simulink model "FSAC2021"  (R2014a)
settings: Solver=FixedStepDiscrete  StartTime=0.0  StopTime=inf  FixedStep=0.0005  RelTol=1e-3
model workspace (MAT data in the model file):
  MCOS : class17 (value not decoded)
  MCOS : class17 (value not decoded)
  MCOS : class17 (value not decoded)
  MCOS : class17 (value not decoded)
  MCOS : class17 (value not decoded)
  MCOS : class17 (value not decoded)
  MCOS : class17 (value not decoded)
  MCOS : class17 (value not decoded)
  MCOS : class17 (value not decoded)
  MCOS : class17 (value not decoded)
  MCOS : class17 (value not decoded)
  MCOS : class17 (value not decoded)
  MCOS : class17 (value not decoded)
  MCOS : class17 (value not decoded)
  MCOS : class17 (value not decoded)
  MCOS : class17 (value not decoded)
  MCOS : class17 (value not decoded)
  MCOS : class17 (value not decoded)
  MCOS : class17 (value not decoded)
  BUZZER_START = 1
  MCOS : class17 (value not decoded)
  MCOS : class17 (value not decoded)
  MCOS : class17 (value not decoded)
  MCOS : class17 (value not decoded)
  MCOS : class17 (value not decoded)
  MCOS : class17 (value not decoded)
  MCOS : class17 (value not decoded)
  MCOS : class17 (value not decoded)
  MCOS : class17 (value not decoded)
  MCOS : class17 (value not decoded)
  MCOS : class17 (value not decoded)
  MCOS : class17 (value not decoded)
  MCOS : class17 (value not decoded)
  MCOS : class17 (value not decoded)
  MCOS : class17 (value not decoded)
  MCOS : class17 (value not decoded)
  MCOS : class17 (value not decoded)
  MCOS : class17 (value not decoded)
  MCOS : class17 (value not decoded)
  MCOS : class17 (value not decoded)
  MCOS : class17 (value not decoded)
  MCOS : class17 (value not decoded)
  MCOS : class17 (value not decoded)
  MCOS : class17 (value not decoded)
  MCOS : class17 (value not decoded)
  MCOS : class17 (value not decoded)
  MCOS : class17 (value not decoded)
  MCOS : class17 (value not decoded)
  MCOS : class17 (value not decoded)
  MCOS : class17 (value not decoded)
  MCOS : class17 (value not decoded)
  MCOS : class17 (value not decoded)
  MCOS : class17 (value not decoded)
  MCOS : class17 (value not decoded)
  MCOS : class17 (value not decoded)
  MCOS : class17 (value not decoded)
  MCOS : class17 (value not decoded)
  MCOS : class17 (value not decoded)
  Brake = 11
  MCOS : class17 (value not decoded)
  MCOS : class17 (value not decoded)
  MCOS : class17 (value not decoded)
  MCOS : class17 (value not decoded)
  MCOS : class17 (value not decoded)
  MCOS : class17 (value not decoded)
  MCOS : class17 (value not decoded)
  MCOS : class17 (value not decoded)
  Sensor_Acc_b = 101.85
  Sensor_Acc_k = -0.0185
  Str_Sen_Orig_Angle = -341
  MCOS : class17 (value not decoded)
  Tire_D = 0.47
  T = 0.05
libraries: simulink x396, ec55xxlib x126
(part 6 of 17)

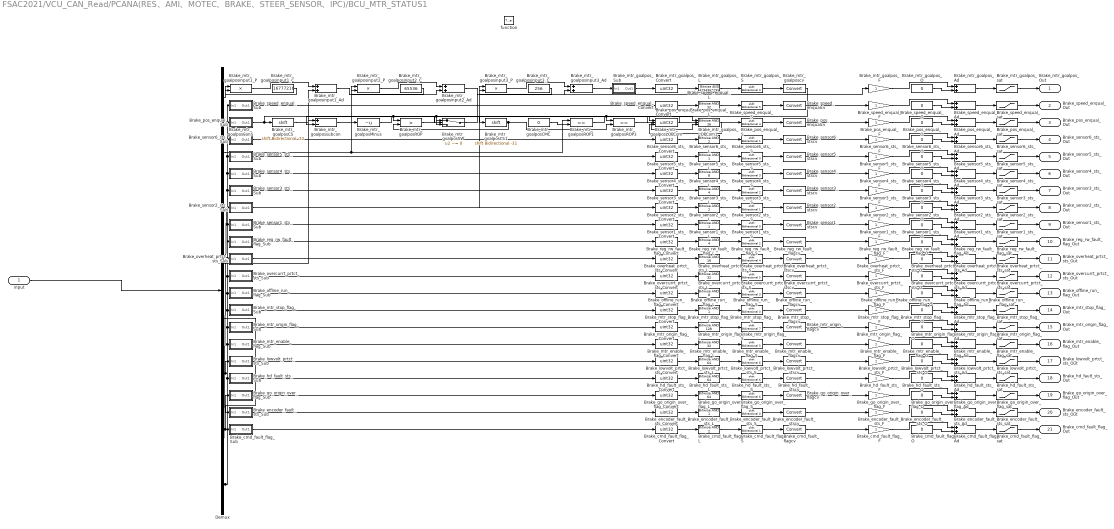
== system FSAC2021/VCU_CAN_Read/PCANA(RES、AMI、MOTEC、BRAKE、STEER_SENSOR、IPC)/BCU_MTR_STATUS1 ==
  input : Inport
  function : TriggerPort  TriggerType=function-call
  Brake_cmd_fault_flag_Ad : Sum
  Brake_cmd_fault_flag_Convert : DataTypeConversion  OutDataTypeStr=uint32
  Brake_cmd_fault_flag_F : Gain
  Brake_cmd_fault_flag_L : simulink/Logic and Bit Operations/Bitwise Operator  logicop=AND  UseBitMask=on  BitMask=2  BitMaskRealWorld=Stored Integer
  Brake_cmd_fault_flag_O : Constant  Value=0  OutDataTypeStr=single
  Brake_cmd_fault_flag_S : ArithShift  BitShiftNumber=1
  Brake_cmd_fault_flag_Sub : Subsystem
  Brake_cmd_fault_flag_sat : Saturate  UpperLimit=1  LowerLimit=0
  Brake_cmd_fault_flagcv : DataTypeConversion
  Brake_encoder_fault_sts_Ad : Sum
  Brake_encoder_fault_sts_Convert : DataTypeConversion  OutDataTypeStr=uint32
  Brake_encoder_fault_sts_F : Gain
  Brake_encoder_fault_sts_L : simulink/Logic and Bit Operations/Bitwise Operator  logicop=AND  UseBitMask=on  BitMask=1  BitMaskRealWorld=Stored Integer
  Brake_encoder_fault_sts_O : Constant  Value=0  OutDataTypeStr=single
  Brake_encoder_fault_sts_S : ArithShift
  Brake_encoder_fault_sts_Sub : Subsystem
  Brake_encoder_fault_sts_sat : Saturate  UpperLimit=1  LowerLimit=0
  Brake_encoder_fault_stscv : DataTypeConversion
  Brake_go_origin_over_flag_Ad : Sum
  Brake_go_origin_over_flag_Convert : DataTypeConversion  OutDataTypeStr=uint32
  Brake_go_origin_over_flag_F : Gain
  Brake_go_origin_over_flag_L : simulink/Logic and Bit Operations/Bitwise Operator  logicop=AND  UseBitMask=on  BitMask=64  BitMaskRealWorld=Stored Integer
  Brake_go_origin_over_flag_O : Constant  Value=0  OutDataTypeStr=single
  Brake_go_origin_over_flag_S : ArithShift  BitShiftNumber=6
  Brake_go_origin_over_flag_Sub : Subsystem
  Brake_go_origin_over_flag_sat : Saturate  UpperLimit=1  LowerLimit=0
  Brake_go_origin_over_flagcv : DataTypeConversion
  Brake_hd_fault_sts_Ad : Sum
  Brake_hd_fault_sts_Convert : DataTypeConversion  OutDataTypeStr=uint32
  Brake_hd_fault_sts_F : Gain
  Brake_hd_fault_sts_L : simulink/Logic and Bit Operations/Bitwise Operator  logicop=AND  UseBitMask=on  BitMask=64  BitMaskRealWorld=Stored Integer
  Brake_hd_fault_sts_O : Constant  Value=0  OutDataTypeStr=single
  Brake_hd_fault_sts_S : ArithShift  BitShiftNumber=6
  Brake_hd_fault_sts_Sub : Subsystem
  Brake_hd_fault_sts_sat : Saturate  UpperLimit=1  LowerLimit=0
  Brake_hd_fault_stscv : DataTypeConversion
  Brake_lowvolt_prtct_sts_Ad : Sum
  Brake_lowvolt_prtct_sts_Convert : DataTypeConversion  OutDataTypeStr=uint32
  Brake_lowvolt_prtct_sts_F : Gain
  Brake_lowvolt_prtct_sts_L : simulink/Logic and Bit Operations/Bitwise Operator  logicop=AND  UseBitMask=on  BitMask=64  BitMaskRealWorld=Stored Integer
  Brake_lowvolt_prtct_sts_O : Constant  Value=0  OutDataTypeStr=single
  Brake_lowvolt_prtct_sts_S : ArithShift  BitShiftNumber=6
  Brake_lowvolt_prtct_sts_Sub : Subsystem
  Brake_lowvolt_prtct_sts_sat : Saturate  UpperLimit=1  LowerLimit=0
  Brake_lowvolt_prtct_stscv : DataTypeConversion
  Brake_mtr_enable_flag_Ad : Sum
  Brake_mtr_enable_flag_Convert : DataTypeConversion  OutDataTypeStr=uint32
  Brake_mtr_enable_flag_F : Gain
  Brake_mtr_enable_flag_L : simulink/Logic and Bit Operations/Bitwise Operator  logicop=AND  UseBitMask=on  BitMask=32  BitMaskRealWorld=Stored Integer
  Brake_mtr_enable_flag_O : Constant  Value=0  OutDataTypeStr=single
  Brake_mtr_enable_flag_S : ArithShift  BitShiftNumber=5
  Brake_mtr_enable_flag_Sub : Subsystem
  Brake_mtr_enable_flag_sat : Saturate  UpperLimit=1  LowerLimit=0
  Brake_mtr_enable_flagcv : DataTypeConversion
  Brake_mtr_goalposCMC : Constant  Value=0
  Brake_mtr_goalposCS : ArithShift  BitShiftNumber=-32
  Brake_mtr_goalposCS1 : ArithShift  BitShiftNumber=-31
  Brake_mtr_goalposConS : Constant  OutDataTypeStr=single
  Brake_mtr_goalposLOPCom : Logic  Operator=OR  AllPortsSameDT=off  OutDataTypeStr=boolean
  Brake_mtr_goalposMinus : UnaryMinus
  Brake_mtr_goalposROP : RelationalOperator  Operator=>  OutDataTypeStr=boolean
  Brake_mtr_goalposROP1 : RelationalOperator  Operator===  OutDataTypeStr=boolean
  Brake_mtr_goalposROP3 : RelationalOperator  Operator===  OutDataTypeStr=boolean
  Brake_mtr_goalposSW : Switch  Criteria=u2 ~= 0
  Brake_mtr_goalpos_Ad : Sum
  Brake_mtr_goalpos_Convert : DataTypeConversion  OutDataTypeStr=uint32
  Brake_mtr_goalpos_F : Gain
  Brake_mtr_goalpos_L : simulink/Logic and Bit Operations/Bitwise Operator  logicop=AND  UseBitMask=on  BitMask=4294967295  BitMaskRealWorld=Stored Integer
  Brake_mtr_goalpos_LOPCom1 : Logic  AllPortsSameDT=off  OutDataTypeStr=boolean
  Brake_mtr_goalpos_O : Constant  Value=0  OutDataTypeStr=single
  Brake_mtr_goalpos_S : ArithShift
  Brake_mtr_goalpos_Sub : Subsystem
  Brake_mtr_goalpos_sat : Saturate  UpperLimit=2147483647  LowerLimit=-2147483648
  Brake_mtr_goalposcv : DataTypeConversion
  Brake_mtr_goalposinput1_Ad : Sum
  Brake_mtr_goalposinput1_C : Constant  Value=16777216
  Brake_mtr_goalposinput1_P : Product
  Brake_mtr_goalposinput2_Ad : Sum
  Brake_mtr_goalposinput2_C : Constant  Value=65536
  Brake_mtr_goalposinput2_P : Product
  Brake_mtr_goalposinput3_Ad : Sum
  Brake_mtr_goalposinput3_C : Constant  Value=256
  Brake_mtr_goalposinput3_P : Product
  Brake_mtr_goalpossubcon : Sum  Inputs=+-
  Brake_mtr_origin_flag_Ad : Sum
  Brake_mtr_origin_flag_Convert : DataTypeConversion  OutDataTypeStr=uint32
  Brake_mtr_origin_flag_F : Gain
  Brake_mtr_origin_flag_L : simulink/Logic and Bit Operations/Bitwise Operator  logicop=AND  UseBitMask=on  BitMask=128  BitMaskRealWorld=Stored Integer
  Brake_mtr_origin_flag_O : Constant  Value=0  OutDataTypeStr=single
  Brake_mtr_origin_flag_S : ArithShift  BitShiftNumber=7
  Brake_mtr_origin_flag_Sub : Subsystem
  Brake_mtr_origin_flag_sat : Saturate  UpperLimit=1  LowerLimit=0
  Brake_mtr_origin_flagcv : DataTypeConversion
  Brake_mtr_stop_flag_Ad : Sum
  Brake_mtr_stop_flag_Convert : DataTypeConversion  OutDataTypeStr=uint32
  Brake_mtr_stop_flag_F : Gain
  Brake_mtr_stop_flag_L : simulink/Logic and Bit Operations/Bitwise Operator  logicop=AND  UseBitMask=on  BitMask=1  BitMaskRealWorld=Stored Integer
  Brake_mtr_stop_flag_O : Constant  Value=0  OutDataTypeStr=single
  Brake_mtr_stop_flag_S : ArithShift
  Brake_mtr_stop_flag_Sub : Subsystem
  Brake_mtr_stop_flag_sat : Saturate  UpperLimit=1  LowerLimit=0
  Brake_mtr_stop_flagcv : DataTypeConversion
  Brake_offline_run_flag_Ad : Sum
  Brake_offline_run_flag_Convert : DataTypeConversion  OutDataTypeStr=uint32
  Brake_offline_run_flag_F : Gain
  Brake_offline_run_flag_L : simulink/Logic and Bit Operations/Bitwise Operator  logicop=AND  UseBitMask=on  BitMask=8  BitMaskRealWorld=Stored Integer
  Brake_offline_run_flag_O : Constant  Value=0  OutDataTypeStr=single
  Brake_offline_run_flag_S : ArithShift  BitShiftNumber=3
  Brake_offline_run_flag_Sub : Subsystem
  Brake_offline_run_flag_sat : Saturate  UpperLimit=1  LowerLimit=0
  Brake_offline_run_flagcv : DataTypeConversion
  Brake_overcurrt_prtct_sts_Ad : Sum
  Brake_overcurrt_prtct_sts_Convert : DataTypeConversion  OutDataTypeStr=uint32
  Brake_overcurrt_prtct_sts_F : Gain
  Brake_overcurrt_prtct_sts_L : simulink/Logic and Bit Operations/Bitwise Operator  logicop=AND  UseBitMask=on  BitMask=32  BitMaskRealWorld=Stored Integer
  Brake_overcurrt_prtct_sts_O : Constant  Value=0  OutDataTypeStr=single
  Brake_overcurrt_prtct_sts_S : ArithShift  BitShiftNumber=5
  Brake_overcurrt_prtct_sts_Sub : Subsystem
  Brake_overcurrt_prtct_sts_sat : Saturate  UpperLimit=1  LowerLimit=0
  Brake_overcurrt_prtct_stscv : DataTypeConversion
  Brake_overheat_prtct_sts_Ad : Sum
  Brake_overheat_prtct_sts_Convert : DataTypeConversion  OutDataTypeStr=uint32
  Brake_overheat_prtct_sts_F : Gain
  Brake_overheat_prtct_sts_L : simulink/Logic and Bit Operations/Bitwise Operator  logicop=AND  UseBitMask=on  BitMask=16  BitMaskRealWorld=Stored Integer
  Brake_overheat_prtct_sts_O : Constant  Value=0  OutDataTypeStr=single
  Brake_overheat_prtct_sts_S : ArithShift  BitShiftNumber=4
  Brake_overheat_prtct_sts_Sub : Subsystem
  Brake_overheat_prtct_sts_sat : Saturate  UpperLimit=1  LowerLimit=0
  Brake_overheat_prtct_stscv : DataTypeConversion
  Brake_pos_enqual_Ad : Sum
  Brake_pos_enqual_Convert : DataTypeConversion  OutDataTypeStr=uint32
  Brake_pos_enqual_F : Gain
  Brake_pos_enqual_L : simulink/Logic and Bit Operations/Bitwise Operator  logicop=AND  UseBitMask=on  BitMask=16  BitMaskRealWorld=Stored Integer
  Brake_pos_enqual_O : Constant  Value=0  OutDataTypeStr=single
  Brake_pos_enqual_S : ArithShift  BitShiftNumber=4
  Brake_pos_enqual_Sub : Subsystem
  Brake_pos_enqual_sat : Saturate  UpperLimit=1  LowerLimit=0
  Brake_pos_enqualcv : DataTypeConversion
  Brake_reg_rw_fault_flag_Ad : Sum
  Brake_reg_rw_fault_flag_Convert : DataTypeConversion  OutDataTypeStr=uint32
  Brake_reg_rw_fault_flag_F : Gain
  Brake_reg_rw_fault_flag_L : simulink/Logic and Bit Operations/Bitwise Operator  logicop=AND  UseBitMask=on  BitMask=4  BitMaskRealWorld=Stored Integer
  Brake_reg_rw_fault_flag_O : Constant  Value=0  OutDataTypeStr=single
  Brake_reg_rw_fault_flag_S : ArithShift  BitShiftNumber=2
  Brake_reg_rw_fault_flag_Sub : Subsystem
  Brake_reg_rw_fault_flag_sat : Saturate  UpperLimit=1  LowerLimit=0
  Brake_reg_rw_fault_flagcv : DataTypeConversion
  Brake_sensor1_sts_Ad : Sum
  Brake_sensor1_sts_Convert : DataTypeConversion  OutDataTypeStr=uint32
  Brake_sensor1_sts_F : Gain
  Brake_sensor1_sts_L : simulink/Logic and Bit Operations/Bitwise Operator  logicop=AND  UseBitMask=on  BitMask=1  BitMaskRealWorld=Stored Integer
  Brake_sensor1_sts_O : Constant  Value=0  OutDataTypeStr=single
  Brake_sensor1_sts_S : ArithShift
  Brake_sensor1_sts_Sub : Subsystem
  Brake_sensor1_sts_sat : Saturate  UpperLimit=1  LowerLimit=0
  Brake_sensor1_stscv : DataTypeConversion
  Brake_sensor2_sts_Ad : Sum
  Brake_sensor2_sts_Convert : DataTypeConversion  OutDataTypeStr=uint32
  Brake_sensor2_sts_F : Gain
  Brake_sensor2_sts_L : simulink/Logic and Bit Operations/Bitwise Operator  logicop=AND  UseBitMask=on  BitMask=2  BitMaskRealWorld=Stored Integer
  Brake_sensor2_sts_O : Constant  Value=0  OutDataTypeStr=single
  Brake_sensor2_sts_S : ArithShift  BitShiftNumber=1
  Brake_sensor2_sts_Sub : Subsystem
  Brake_sensor2_sts_sat : Saturate  UpperLimit=1  LowerLimit=0
  Brake_sensor2_stscv : DataTypeConversion
  Brake_sensor3_sts_Ad : Sum
  Brake_sensor3_sts_Convert : DataTypeConversion  OutDataTypeStr=uint32
  Brake_sensor3_sts_F : Gain
  Brake_sensor3_sts_L : simulink/Logic and Bit Operations/Bitwise Operator  logicop=AND  UseBitMask=on  BitMask=4  BitMaskRealWorld=Stored Integer
  Brake_sensor3_sts_O : Constant  Value=0  OutDataTypeStr=single
  Brake_sensor3_sts_S : ArithShift  BitShiftNumber=2
  Brake_sensor3_sts_Sub : Subsystem
  Brake_sensor3_sts_sat : Saturate  UpperLimit=1  LowerLimit=0
  Brake_sensor3_stscv : DataTypeConversion
  Brake_sensor4_sts_Ad : Sum
  Brake_sensor4_sts_Convert : DataTypeConversion  OutDataTypeStr=uint32
  Brake_sensor4_sts_F : Gain
  Brake_sensor4_sts_L : simulink/Logic and Bit Operations/Bitwise Operator  logicop=AND  UseBitMask=on  BitMask=8  BitMaskRealWorld=Stored Integer
  Brake_sensor4_sts_O : Constant  Value=0  OutDataTypeStr=single
  Brake_sensor4_sts_S : ArithShift  BitShiftNumber=3
  Brake_sensor4_sts_Sub : Subsystem
  Brake_sensor4_sts_sat : Saturate  UpperLimit=1  LowerLimit=0
  Brake_sensor4_stscv : DataTypeConversion
  Brake_sensor5_sts_Ad : Sum
  Brake_sensor5_sts_Convert : DataTypeConversion  OutDataTypeStr=uint32
  Brake_sensor5_sts_F : Gain
  Brake_sensor5_sts_L : simulink/Logic and Bit Operations/Bitwise Operator  logicop=AND  UseBitMask=on  BitMask=1  BitMaskRealWorld=Stored Integer
  Brake_sensor5_sts_O : Constant  Value=0  OutDataTypeStr=single
  Brake_sensor5_sts_S : ArithShift
  Brake_sensor5_sts_Sub : Subsystem
  Brake_sensor5_sts_sat : Saturate  UpperLimit=1  LowerLimit=0
  Brake_sensor5_stscv : DataTypeConversion
  Brake_sensor6_sts_Ad : Sum
  Brake_sensor6_sts_Convert : DataTypeConversion  OutDataTypeStr=uint32
  Brake_sensor6_sts_F : Gain
  Brake_sensor6_sts_L : simulink/Logic and Bit Operations/Bitwise Operator  logicop=AND  UseBitMask=on  BitMask=2  BitMaskRealWorld=Stored Integer
  Brake_sensor6_sts_O : Constant  Value=0  OutDataTypeStr=single
  Brake_sensor6_sts_S : ArithShift  BitShiftNumber=1
  Brake_sensor6_sts_Sub : Subsystem
  Brake_sensor6_sts_sat : Saturate  UpperLimit=1  LowerLimit=0
  Brake_sensor6_stscv : DataTypeConversion
  Brake_speed_enqual_Ad : Sum
  Brake_speed_enqual_Convert : DataTypeConversion  OutDataTypeStr=uint32
  Brake_speed_enqual_F : Gain
  Brake_speed_enqual_L : simulink/Logic and Bit Operations/Bitwise Operator  logicop=AND  UseBitMask=on  BitMask=32  BitMaskRealWorld=Stored Integer
  Brake_speed_enqual_O : Constant  Value=0  OutDataTypeStr=single
  Brake_speed_enqual_S : ArithShift  BitShiftNumber=5
  Brake_speed_enqual_Sub : Subsystem
  Brake_speed_enqual_sat : Saturate  UpperLimit=1  LowerLimit=0
  Brake_speed_enqualcv : DataTypeConversion
  Demux : Demux  Outputs=8
  Brake_mtr_goalpos_Out : Outport
  Brake_speed_enqual_Out : Outport  Port=2
  Brake_pos_enqual_Out : Outport  Port=3
  Brake_sensor6_sts_Out : Outport  Port=4
  Brake_sensor5_sts_Out : Outport  Port=5
  Brake_sensor4_sts_Out : Outport  Port=6
  Brake_sensor3_sts_Out : Outport  Port=7
  Brake_sensor2_sts_Out : Outport  Port=8
  Brake_sensor1_sts_Out : Outport  Port=9
  Brake_reg_rw_fault_flag_Out : Outport  Port=10
  Brake_overheat_prtct_sts_Out : Outport  Port=11
  Brake_overcurrt_prtct_sts_Out : Outport  Port=12
  Brake_offline_run_flag_Out : Outport  Port=13
  Brake_mtr_stop_flag_Out : Outport  Port=14
  Brake_mtr_origin_flag_Out : Outport  Port=15
  Brake_mtr_enable_flag_Out : Outport  Port=16
  Brake_lowvolt_prtct_sts_Out : Outport  Port=17
  Brake_hd_fault_sts_Out : Outport  Port=18
  Brake_go_origin_over_flag_Out : Outport  Port=19
  Brake_encoder_fault_sts_Out : Outport  Port=20
  Brake_cmd_fault_flag_Out : Outport  Port=21
  wires:
  Brake_mtr_goalpos_F/1 -> Brake_mtr_goalpos_Ad/1
  Brake_mtr_goalpos_O/1 -> Brake_mtr_goalpos_Ad/2
  Brake_mtr_goalpos_Ad/1 -> Brake_mtr_goalpos_sat/1
  Brake_mtr_goalpos_sat/1 -> Brake_mtr_goalpos_Out/1
  Demux/1 -> Brake_mtr_goalposinput1_P/1
  Brake_mtr_goalposinput1_C/1 -> Brake_mtr_goalposinput1_P/2
  Brake_mtr_goalposinput1_P/1 -> Brake_mtr_goalposinput1_Ad/1
  Demux/4 -> Brake_mtr_goalposinput1_Ad/2
  Demux/2 -> Brake_mtr_goalposinput2_P/1, Brake_mtr_goalposROP1/1
  Brake_mtr_goalposinput2_C/1 -> Brake_mtr_goalposinput2_P/2
  Brake_mtr_goalposinput2_P/1 -> Brake_mtr_goalposinput2_Ad/1
  Brake_mtr_goalposinput1_Ad/1 -> Brake_mtr_goalposinput2_Ad/2
  Demux/3 -> Brake_mtr_goalposinput3_P/1
  Brake_mtr_goalposinput3_C/1 -> Brake_mtr_goalposinput3_P/2
  Brake_mtr_goalposinput3_P/1 -> Brake_mtr_goalposinput3_Ad/1
  Brake_mtr_goalposinput2_Ad/1 -> Brake_mtr_goalposinput3_Ad/2
  Brake_mtr_goalposinput3_Ad/1 -> Brake_mtr_goalpos_Sub/1(In1)
  Brake_mtr_goalpos_Sub/1(Out1) -> Brake_mtr_goalpos_Convert/1
  Brake_mtr_goalpos_Convert/1 -> Brake_mtr_goalpos_L/1
  Brake_mtr_goalpos_L/1 -> Brake_mtr_goalpos_S/1
  Brake_mtr_goalpos_S/1 -> Brake_mtr_goalposcv/1
  Brake_mtr_goalposcv/1 -> Brake_mtr_goalposROP/1, Brake_mtr_goalpossubcon/2, Brake_mtr_goalposSW/3, Brake_mtr_goalposROP3/1
  Brake_mtr_goalposConS/1 -> Brake_mtr_goalposCS/1, Brake_mtr_goalposCS1/1
  Brake_mtr_goalposCS1/1 -> Brake_mtr_goalposROP/2, Brake_mtr_goalposROP3/2
  Brake_mtr_goalposCS/1 -> Brake_mtr_goalpossubcon/1
  Brake_mtr_goalpossubcon/1 -> Brake_mtr_goalposMinus/1
  Brake_mtr_goalposMinus/1 -> Brake_mtr_goalposSW/1
  Brake_mtr_goalposSW/1 -> Brake_mtr_goalpos_F/1
  Brake_mtr_goalposROP1/1 -> Brake_mtr_goalpos_LOPCom1/1
  Brake_mtr_goalposROP3/1 -> Brake_mtr_goalpos_LOPCom1/2
  Brake_mtr_goalpos_LOPCom1/1 -> Brake_mtr_goalposLOPCom/2
  Brake_mtr_goalposROP/1 -> Brake_mtr_goalposLOPCom/1
  Brake_mtr_goalposLOPCom/1 -> Brake_mtr_goalposSW/2
  Brake_mtr_goalposCMC/1 -> Brake_mtr_goalposROP1/2
  Brake_speed_enqual_F/1 -> Brake_speed_enqual_Ad/1
  Brake_speed_enqual_O/1 -> Brake_speed_enqual_Ad/2
  Brake_speed_enqual_Ad/1 -> Brake_speed_enqual_sat/1
  Brake_speed_enqual_sat/1 -> Brake_speed_enqual_Out/1
  Demux/8 -> Brake_speed_enqual_Sub/1(In1), Brake_pos_enqual_Sub/1(In1), Brake_sensor4_sts_Sub/1(In1), Brake_sensor3_sts_Sub/1(In1), Brake_sensor1_sts_Sub/1(In1), Brake_mtr_origin_flag_Sub/1(In1), Brake_hd_fault_sts_Sub/1(In1), Brake_sensor2_sts_Sub/1(In1)
  Brake_speed_enqual_Sub/1(Out1) -> Brake_speed_enqual_Convert/1
  Brake_speed_enqual_Convert/1 -> Brake_speed_enqual_L/1
  Brake_speed_enqual_L/1 -> Brake_speed_enqual_S/1
  Brake_speed_enqual_S/1 -> Brake_speed_enqualcv/1
  Brake_speed_enqualcv/1 -> Brake_speed_enqual_F/1
  Brake_pos_enqual_F/1 -> Brake_pos_enqual_Ad/1
  Brake_pos_enqual_O/1 -> Brake_pos_enqual_Ad/2
  Brake_pos_enqual_Ad/1 -> Brake_pos_enqual_sat/1
  Brake_pos_enqual_sat/1 -> Brake_pos_enqual_Out/1
  Brake_pos_enqual_Sub/1(Out1) -> Brake_pos_enqual_Convert/1
  Brake_pos_enqual_Convert/1 -> Brake_pos_enqual_L/1
  Brake_pos_enqual_L/1 -> Brake_pos_enqual_S/1
  Brake_pos_enqual_S/1 -> Brake_pos_enqualcv/1
  Brake_pos_enqualcv/1 -> Brake_pos_enqual_F/1
  Brake_sensor6_sts_F/1 -> Brake_sensor6_sts_Ad/1
  Brake_sensor6_sts_O/1 -> Brake_sensor6_sts_Ad/2
  Brake_sensor6_sts_Ad/1 -> Brake_sensor6_sts_sat/1
  Brake_sensor6_sts_sat/1 -> Brake_sensor6_sts_Out/1
  Demux/6 -> Brake_sensor6_sts_Sub/1(In1), Brake_sensor5_sts_Sub/1(In1), Brake_overheat_prtct_sts_Sub/1(In1), Brake_overcurrt_prtct_sts_Sub/1(In1), Brake_lowvolt_prtct_sts_Sub/1(In1)
  Brake_sensor6_sts_Sub/1(Out1) -> Brake_sensor6_sts_Convert/1
  Brake_sensor6_sts_Convert/1 -> Brake_sensor6_sts_L/1
  Brake_sensor6_sts_L/1 -> Brake_sensor6_sts_S/1
  Brake_sensor6_sts_S/1 -> Brake_sensor6_stscv/1
  Brake_sensor6_stscv/1 -> Brake_sensor6_sts_F/1
  Brake_sensor5_sts_F/1 -> Brake_sensor5_sts_Ad/1
  Brake_sensor5_sts_O/1 -> Brake_sensor5_sts_Ad/2
  Brake_sensor5_sts_Ad/1 -> Brake_sensor5_sts_sat/1
  Brake_sensor5_sts_sat/1 -> Brake_sensor5_sts_Out/1
  Brake_sensor5_sts_Sub/1(Out1) -> Brake_sensor5_sts_Convert/1
  Brake_sensor5_sts_Convert/1 -> Brake_sensor5_sts_L/1
  Brake_sensor5_sts_L/1 -> Brake_sensor5_sts_S/1
  Brake_sensor5_sts_S/1 -> Brake_sensor5_stscv/1
  Brake_sensor5_stscv/1 -> Brake_sensor5_sts_F/1
  Brake_sensor4_sts_F/1 -> Brake_sensor4_sts_Ad/1
  Brake_sensor4_sts_O/1 -> Brake_sensor4_sts_Ad/2
  Brake_sensor4_sts_Ad/1 -> Brake_sensor4_sts_sat/1
  Brake_sensor4_sts_sat/1 -> Brake_sensor4_sts_Out/1
  Brake_sensor4_sts_Sub/1(Out1) -> Brake_sensor4_sts_Convert/1
  Brake_sensor4_sts_Convert/1 -> Brake_sensor4_sts_L/1
  Brake_sensor4_sts_L/1 -> Brake_sensor4_sts_S/1
  Brake_sensor4_sts_S/1 -> Brake_sensor4_stscv/1
  Brake_sensor4_stscv/1 -> Brake_sensor4_sts_F/1
  Brake_sensor3_sts_F/1 -> Brake_sensor3_sts_Ad/1
  Brake_sensor3_sts_O/1 -> Brake_sensor3_sts_Ad/2
  Brake_sensor3_sts_Ad/1 -> Brake_sensor3_sts_sat/1
  Brake_sensor3_sts_sat/1 -> Brake_sensor3_sts_Out/1
  Brake_sensor3_sts_Sub/1(Out1) -> Brake_sensor3_sts_Convert/1
  Brake_sensor3_sts_Convert/1 -> Brake_sensor3_sts_L/1
  Brake_sensor3_sts_L/1 -> Brake_sensor3_sts_S/1
  Brake_sensor3_sts_S/1 -> Brake_sensor3_stscv/1
  Brake_sensor3_stscv/1 -> Brake_sensor3_sts_F/1
  Brake_sensor2_sts_F/1 -> Brake_sensor2_sts_Ad/1
  Brake_sensor2_sts_O/1 -> Brake_sensor2_sts_Ad/2
  Brake_sensor2_sts_Ad/1 -> Brake_sensor2_sts_sat/1
  Brake_sensor2_sts_sat/1 -> Brake_sensor2_sts_Out/1
  Brake_sensor2_sts_Sub/1(Out1) -> Brake_sensor2_sts_Convert/1
  Brake_sensor2_sts_Convert/1 -> Brake_sensor2_sts_L/1
  Brake_sensor2_sts_L/1 -> Brake_sensor2_sts_S/1
  Brake_sensor2_sts_S/1 -> Brake_sensor2_stscv/1
  Brake_sensor2_stscv/1 -> Brake_sensor2_sts_F/1
  Brake_sensor1_sts_F/1 -> Brake_sensor1_sts_Ad/1
  Brake_sensor1_sts_O/1 -> Brake_sensor1_sts_Ad/2
  Brake_sensor1_sts_Ad/1 -> Brake_sensor1_sts_sat/1
  Brake_sensor1_sts_sat/1 -> Brake_sensor1_sts_Out/1
  Brake_sensor1_sts_Sub/1(Out1) -> Brake_sensor1_sts_Convert/1
  Brake_sensor1_sts_Convert/1 -> Brake_sensor1_sts_L/1
  Brake_sensor1_sts_L/1 -> Brake_sensor1_sts_S/1
  Brake_sensor1_sts_S/1 -> Brake_sensor1_stscv/1
  Brake_sensor1_stscv/1 -> Brake_sensor1_sts_F/1
  Brake_reg_rw_fault_flag_F/1 -> Brake_reg_rw_fault_flag_Ad/1
  Brake_reg_rw_fault_flag_O/1 -> Brake_reg_rw_fault_flag_Ad/2
  Brake_reg_rw_fault_flag_Ad/1 -> Brake_reg_rw_fault_flag_sat/1
  Brake_reg_rw_fault_flag_sat/1 -> Brake_reg_rw_fault_flag_Out/1
  Demux/7 -> Brake_reg_rw_fault_flag_Sub/1(In1), Brake_offline_run_flag_Sub/1(In1), Brake_mtr_stop_flag_Sub/1(In1), Brake_mtr_enable_flag_Sub/1(In1), Brake_go_origin_over_flag_Sub/1(In1), Brake_cmd_fault_flag_Sub/1(In1)
  Brake_reg_rw_fault_flag_Sub/1(Out1) -> Brake_reg_rw_fault_flag_Convert/1
  Brake_reg_rw_fault_flag_Convert/1 -> Brake_reg_rw_fault_flag_L/1
  Brake_reg_rw_fault_flag_L/1 -> Brake_reg_rw_fault_flag_S/1
  Brake_reg_rw_fault_flag_S/1 -> Brake_reg_rw_fault_flagcv/1
  Brake_reg_rw_fault_flagcv/1 -> Brake_reg_rw_fault_flag_F/1
  Brake_overheat_prtct_sts_F/1 -> Brake_overheat_prtct_sts_Ad/1
  Brake_overheat_prtct_sts_O/1 -> Brake_overheat_prtct_sts_Ad/2
  Brake_overheat_prtct_sts_Ad/1 -> Brake_overheat_prtct_sts_sat/1
  Brake_overheat_prtct_sts_sat/1 -> Brake_overheat_prtct_sts_Out/1
  Brake_overheat_prtct_sts_Sub/1(Out1) -> Brake_overheat_prtct_sts_Convert/1
  Brake_overheat_prtct_sts_Convert/1 -> Brake_overheat_prtct_sts_L/1
  Brake_overheat_prtct_sts_L/1 -> Brake_overheat_prtct_sts_S/1
  Brake_overheat_prtct_sts_S/1 -> Brake_overheat_prtct_stscv/1
  Brake_overheat_prtct_stscv/1 -> Brake_overheat_prtct_sts_F/1
  Brake_overcurrt_prtct_sts_F/1 -> Brake_overcurrt_prtct_sts_Ad/1
  Brake_overcurrt_prtct_sts_O/1 -> Brake_overcurrt_prtct_sts_Ad/2
  Brake_overcurrt_prtct_sts_Ad/1 -> Brake_overcurrt_prtct_sts_sat/1
  Brake_overcurrt_prtct_sts_sat/1 -> Brake_overcurrt_prtct_sts_Out/1
  Brake_overcurrt_prtct_sts_Sub/1(Out1) -> Brake_overcurrt_prtct_sts_Convert/1
  Brake_overcurrt_prtct_sts_Convert/1 -> Brake_overcurrt_prtct_sts_L/1
  Brake_overcurrt_prtct_sts_L/1 -> Brake_overcurrt_prtct_sts_S/1
  Brake_overcurrt_prtct_sts_S/1 -> Brake_overcurrt_prtct_stscv/1
  Brake_overcurrt_prtct_stscv/1 -> Brake_overcurrt_prtct_sts_F/1
  Brake_offline_run_flag_F/1 -> Brake_offline_run_flag_Ad/1
  Brake_offline_run_flag_O/1 -> Brake_offline_run_flag_Ad/2
  Brake_offline_run_flag_Ad/1 -> Brake_offline_run_flag_sat/1
  Brake_offline_run_flag_sat/1 -> Brake_offline_run_flag_Out/1
  Brake_offline_run_flag_Sub/1(Out1) -> Brake_offline_run_flag_Convert/1
  Brake_offline_run_flag_Convert/1 -> Brake_offline_run_flag_L/1
  Brake_offline_run_flag_L/1 -> Brake_offline_run_flag_S/1
  Brake_offline_run_flag_S/1 -> Brake_offline_run_flagcv/1
  Brake_offline_run_flagcv/1 -> Brake_offline_run_flag_F/1
  Brake_mtr_stop_flag_F/1 -> Brake_mtr_stop_flag_Ad/1
  Brake_mtr_stop_flag_O/1 -> Brake_mtr_stop_flag_Ad/2
  Brake_mtr_stop_flag_Ad/1 -> Brake_mtr_stop_flag_sat/1
  Brake_mtr_stop_flag_sat/1 -> Brake_mtr_stop_flag_Out/1
  Brake_mtr_stop_flag_Sub/1(Out1) -> Brake_mtr_stop_flag_Convert/1
  Brake_mtr_stop_flag_Convert/1 -> Brake_mtr_stop_flag_L/1
  Brake_mtr_stop_flag_L/1 -> Brake_mtr_stop_flag_S/1
  Brake_mtr_stop_flag_S/1 -> Brake_mtr_stop_flagcv/1
  Brake_mtr_stop_flagcv/1 -> Brake_mtr_stop_flag_F/1
  Brake_mtr_origin_flag_F/1 -> Brake_mtr_origin_flag_Ad/1
  Brake_mtr_origin_flag_O/1 -> Brake_mtr_origin_flag_Ad/2
  Brake_mtr_origin_flag_Ad/1 -> Brake_mtr_origin_flag_sat/1
  Brake_mtr_origin_flag_sat/1 -> Brake_mtr_origin_flag_Out/1
  Brake_mtr_origin_flag_Sub/1(Out1) -> Brake_mtr_origin_flag_Convert/1
  Brake_mtr_origin_flag_Convert/1 -> Brake_mtr_origin_flag_L/1
  Brake_mtr_origin_flag_L/1 -> Brake_mtr_origin_flag_S/1
  Brake_mtr_origin_flag_S/1 -> Brake_mtr_origin_flagcv/1
  Brake_mtr_origin_flagcv/1 -> Brake_mtr_origin_flag_F/1
  Brake_mtr_enable_flag_F/1 -> Brake_mtr_enable_flag_Ad/1
  Brake_mtr_enable_flag_O/1 -> Brake_mtr_enable_flag_Ad/2
  Brake_mtr_enable_flag_Ad/1 -> Brake_mtr_enable_flag_sat/1
  Brake_mtr_enable_flag_sat/1 -> Brake_mtr_enable_flag_Out/1
  Brake_mtr_enable_flag_Sub/1(Out1) -> Brake_mtr_enable_flag_Convert/1
  Brake_mtr_enable_flag_Convert/1 -> Brake_mtr_enable_flag_L/1
  Brake_mtr_enable_flag_L/1 -> Brake_mtr_enable_flag_S/1
  Brake_mtr_enable_flag_S/1 -> Brake_mtr_enable_flagcv/1
  Brake_mtr_enable_flagcv/1 -> Brake_mtr_enable_flag_F/1
  Brake_lowvolt_prtct_sts_F/1 -> Brake_lowvolt_prtct_sts_Ad/1
  Brake_lowvolt_prtct_sts_O/1 -> Brake_lowvolt_prtct_sts_Ad/2
  Brake_lowvolt_prtct_sts_Ad/1 -> Brake_lowvolt_prtct_sts_sat/1
  Brake_lowvolt_prtct_sts_sat/1 -> Brake_lowvolt_prtct_sts_Out/1
  Brake_lowvolt_prtct_sts_Sub/1(Out1) -> Brake_lowvolt_prtct_sts_Convert/1
  Brake_lowvolt_prtct_sts_Convert/1 -> Brake_lowvolt_prtct_sts_L/1
  Brake_lowvolt_prtct_sts_L/1 -> Brake_lowvolt_prtct_sts_S/1
  Brake_lowvolt_prtct_sts_S/1 -> Brake_lowvolt_prtct_stscv/1
  Brake_lowvolt_prtct_stscv/1 -> Brake_lowvolt_prtct_sts_F/1
  Brake_hd_fault_sts_F/1 -> Brake_hd_fault_sts_Ad/1
  Brake_hd_fault_sts_O/1 -> Brake_hd_fault_sts_Ad/2
  Brake_hd_fault_sts_Ad/1 -> Brake_hd_fault_sts_sat/1
  Brake_hd_fault_sts_sat/1 -> Brake_hd_fault_sts_Out/1
  Brake_hd_fault_sts_Sub/1(Out1) -> Brake_hd_fault_sts_Convert/1
  Brake_hd_fault_sts_Convert/1 -> Brake_hd_fault_sts_L/1
  Brake_hd_fault_sts_L/1 -> Brake_hd_fault_sts_S/1
  Brake_hd_fault_sts_S/1 -> Brake_hd_fault_stscv/1
  Brake_hd_fault_stscv/1 -> Brake_hd_fault_sts_F/1
  Brake_go_origin_over_flag_F/1 -> Brake_go_origin_over_flag_Ad/1
  Brake_go_origin_over_flag_O/1 -> Brake_go_origin_over_flag_Ad/2
  Brake_go_origin_over_flag_Ad/1 -> Brake_go_origin_over_flag_sat/1
  Brake_go_origin_over_flag_sat/1 -> Brake_go_origin_over_flag_Out/1
  Brake_go_origin_over_flag_Sub/1(Out1) -> Brake_go_origin_over_flag_Convert/1
  Brake_go_origin_over_flag_Convert/1 -> Brake_go_origin_over_flag_L/1
  Brake_go_origin_over_flag_L/1 -> Brake_go_origin_over_flag_S/1
  Brake_go_origin_over_flag_S/1 -> Brake_go_origin_over_flagcv/1
  Brake_go_origin_over_flagcv/1 -> Brake_go_origin_over_flag_F/1
  Brake_encoder_fault_sts_F/1 -> Brake_encoder_fault_sts_Ad/1
  Brake_encoder_fault_sts_O/1 -> Brake_encoder_fault_sts_Ad/2
  Brake_encoder_fault_sts_Ad/1 -> Brake_encoder_fault_sts_sat/1
  Brake_encoder_fault_sts_sat/1 -> Brake_encoder_fault_sts_Out/1
  Demux/5 -> Brake_encoder_fault_sts_Sub/1(In1)
  Brake_encoder_fault_sts_Sub/1(Out1) -> Brake_encoder_fault_sts_Convert/1
  Brake_encoder_fault_sts_Convert/1 -> Brake_encoder_fault_sts_L/1
  Brake_encoder_fault_sts_L/1 -> Brake_encoder_fault_sts_S/1
  Brake_encoder_fault_sts_S/1 -> Brake_encoder_fault_stscv/1
  Brake_encoder_fault_stscv/1 -> Brake_encoder_fault_sts_F/1
  Brake_cmd_fault_flag_F/1 -> Brake_cmd_fault_flag_Ad/1
  Brake_cmd_fault_flag_O/1 -> Brake_cmd_fault_flag_Ad/2
  Brake_cmd_fault_flag_Ad/1 -> Brake_cmd_fault_flag_sat/1
  Brake_cmd_fault_flag_sat/1 -> Brake_cmd_fault_flag_Out/1
  Brake_cmd_fault_flag_Sub/1(Out1) -> Brake_cmd_fault_flag_Convert/1
  Brake_cmd_fault_flag_Convert/1 -> Brake_cmd_fault_flag_L/1
  Brake_cmd_fault_flag_L/1 -> Brake_cmd_fault_flag_S/1
  Brake_cmd_fault_flag_S/1 -> Brake_cmd_fault_flagcv/1
  Brake_cmd_fault_flagcv/1 -> Brake_cmd_fault_flag_F/1
  input/1 -> Demux/1

== system FSAC2021/VCU_CAN_Read/PCANA(RES、AMI、MOTEC、BRAKE、STEER_SENSOR、IPC)/Heartt ==
  input : Inport
  function : TriggerPort  TriggerType=function-call
  Demux : Demux  Outputs=1
  assi_status_Ad : Sum
  assi_status_Convert : DataTypeConversion  OutDataTypeStr=uint32
  assi_status_F : Gain
  assi_status_L : simulink/Logic and Bit Operations/Bitwise Operator  logicop=AND  UseBitMask=on  BitMask=255  BitMaskRealWorld=Stored Integer
  assi_status_O : Constant  Value=0  OutDataTypeStr=single
  assi_status_S : ArithShift
  assi_status_Sub : Subsystem
  assi_status_sat : Saturate  UpperLimit=255  LowerLimit=0
  assi_statuscv : DataTypeConversion
  assi_status_Out : Outport
  wires:
  assi_status_F/1 -> assi_status_Ad/1
  assi_status_O/1 -> assi_status_Ad/2
  assi_status_Ad/1 -> assi_status_sat/1
  assi_status_sat/1 -> assi_status_Out/1
  Demux/1 -> assi_status_Sub/1(In1)
  assi_status_Sub/1(Out1) -> assi_status_Convert/1
  assi_status_Convert/1 -> assi_status_L/1
  assi_status_L/1 -> assi_status_S/1
  assi_status_S/1 -> assi_statuscv/1
  assi_statuscv/1 -> assi_status_F/1
  input/1 -> Demux/1

== system FSAC2021/VCU_CAN_Read/PCANA(RES、AMI、MOTEC、BRAKE、STEER_SENSOR、IPC)/IPC_CMD1 ==
  input : Inport
  function : TriggerPort  TriggerType=function-call
  Demux : Demux  Outputs=3
  IPC_Acc_Ad : Sum
  IPC_Acc_Convert : DataTypeConversion  OutDataTypeStr=uint32
  IPC_Acc_F : Gain
  IPC_Acc_L : simulink/Logic and Bit Operations/Bitwise Operator  logicop=AND  UseBitMask=on  BitMask=255  BitMaskRealWorld=Stored Integer
  IPC_Acc_O : Constant  Value=0  OutDataTypeStr=single
  IPC_Acc_S : ArithShift
  IPC_Acc_Sub : Subsystem
  IPC_Acc_sat : Saturate  UpperLimit=100  LowerLimit=0
  IPC_Acccv : DataTypeConversion
  IPC_Brk_Ad : Sum
  IPC_Brk_Convert : DataTypeConversion  OutDataTypeStr=uint32
  IPC_Brk_F : Gain
  IPC_Brk_L : simulink/Logic and Bit Operations/Bitwise Operator  logicop=AND  UseBitMask=on  BitMask=255  BitMaskRealWorld=Stored Integer
  IPC_Brk_O : Constant  Value=0  OutDataTypeStr=single
  IPC_Brk_S : ArithShift
  IPC_Brk_Sub : Subsystem
  IPC_Brk_sat : Saturate  UpperLimit=100  LowerLimit=0
  IPC_Brkcv : DataTypeConversion
  IPC_Steer_Ad : Sum
  IPC_Steer_Convert : DataTypeConversion  OutDataTypeStr=uint32
  IPC_Steer_F : Gain
  IPC_Steer_L : simulink/Logic and Bit Operations/Bitwise Operator  logicop=AND  UseBitMask=on  BitMask=255  BitMaskRealWorld=Stored Integer
  IPC_Steer_O : Constant  Value=-120  OutDataTypeStr=single
  IPC_Steer_S : ArithShift
  IPC_Steer_Sub : Subsystem
  IPC_Steer_sat : Saturate  UpperLimit=135  LowerLimit=-120
  IPC_Steercv : DataTypeConversion
  IPC_Steer_Out : Outport
  IPC_Brk_Out : Outport  Port=2
  IPC_Acc_Out : Outport  Port=3
  wires:
  IPC_Steer_F/1 -> IPC_Steer_Ad/1
  IPC_Steer_O/1 -> IPC_Steer_Ad/2
  IPC_Steer_Ad/1 -> IPC_Steer_sat/1
  IPC_Steer_sat/1 -> IPC_Steer_Out/1
  Demux/3 -> IPC_Steer_Sub/1(In1)
  IPC_Steer_Sub/1(Out1) -> IPC_Steer_Convert/1
  IPC_Steer_Convert/1 -> IPC_Steer_L/1
  IPC_Steer_L/1 -> IPC_Steer_S/1
  IPC_Steer_S/1 -> IPC_Steercv/1
  IPC_Steercv/1 -> IPC_Steer_F/1
  IPC_Brk_F/1 -> IPC_Brk_Ad/1
  IPC_Brk_O/1 -> IPC_Brk_Ad/2
  IPC_Brk_Ad/1 -> IPC_Brk_sat/1
  IPC_Brk_sat/1 -> IPC_Brk_Out/1
  Demux/2 -> IPC_Brk_Sub/1(In1)
  IPC_Brk_Sub/1(Out1) -> IPC_Brk_Convert/1
  IPC_Brk_Convert/1 -> IPC_Brk_L/1
  IPC_Brk_L/1 -> IPC_Brk_S/1
  IPC_Brk_S/1 -> IPC_Brkcv/1
  IPC_Brkcv/1 -> IPC_Brk_F/1
  IPC_Acc_F/1 -> IPC_Acc_Ad/1
  IPC_Acc_O/1 -> IPC_Acc_Ad/2
  IPC_Acc_Ad/1 -> IPC_Acc_sat/1
  IPC_Acc_sat/1 -> IPC_Acc_Out/1
  Demux/1 -> IPC_Acc_Sub/1(In1)
  IPC_Acc_Sub/1(Out1) -> IPC_Acc_Convert/1
  IPC_Acc_Convert/1 -> IPC_Acc_L/1
  IPC_Acc_L/1 -> IPC_Acc_S/1
  IPC_Acc_S/1 -> IPC_Acccv/1
  IPC_Acccv/1 -> IPC_Acc_F/1
  input/1 -> Demux/1

== system FSAC2021/VCU_CAN_Read/PCANA(RES、AMI、MOTEC、BRAKE、STEER_SENSOR、IPC)/MOTEC_MOTION  ==
  In1 : Inport
  function : TriggerPort  TriggerType=function-call
  Data Type Conversion1 : DataTypeConversion  OutDataTypeStr=int8
  Data Type Conversion12 : DataTypeConversion  OutDataTypeStr=uint16
  Data Type Conversion14 : DataTypeConversion  OutDataTypeStr=int32
  MOTEC_MOTION : Subsystem
  Motec_Currt_Ang_Out : Outport
  Motec_Currt_Current_Out : Outport  Port=2
  Motec_Currt_Position_Out : Outport  Port=3
  wires:
  MOTEC_MOTION/2(Motec_Currt_Current_Out) -> Data Type Conversion1/1
  MOTEC_MOTION/1(Motec_Currt_Ang_Out) -> Data Type Conversion12/1
  Data Type Conversion12/1 -> Motec_Currt_Ang_Out/1
  Data Type Conversion14/1 -> Motec_Currt_Position_Out/1
  MOTEC_MOTION/3(Motec_Currt_Position_Out) -> Data Type Conversion14/1
  In1/1 -> MOTEC_MOTION/1(input)
  Data Type Conversion1/1 -> Motec_Currt_Current_Out/1

== system FSAC2021/VCU_CAN_Read/PCANA(RES、AMI、MOTEC、BRAKE、STEER_SENSOR、IPC)/STEER_SENSOR_INFO1 ==
  input : Inport
  function : TriggerPort  TriggerType=function-call
  Demux : Demux  Outputs=8
  Str_Sensor_Curr_AngleCS : ArithShift  BitShiftNumber=-16
  Str_Sensor_Curr_AngleCS1 : ArithShift  BitShiftNumber=-15
  Str_Sensor_Curr_AngleConS : Constant  OutDataTypeStr=single
  Str_Sensor_Curr_AngleMinus : UnaryMinus
  Str_Sensor_Curr_AngleROP : RelationalOperator  OutDataTypeStr=boolean
  Str_Sensor_Curr_AngleSW : Switch  Criteria=u2 ~= 0
  Str_Sensor_Curr_Angle_Ad : Sum
  Str_Sensor_Curr_Angle_Convert : DataTypeConversion  OutDataTypeStr=uint32
  Str_Sensor_Curr_Angle_F : Gain  Gain=0.0625
  Str_Sensor_Curr_Angle_L : simulink/Logic and Bit Operations/Bitwise Operator  logicop=AND  UseBitMask=on  BitMask=65535  BitMaskRealWorld=Stored Integer
  Str_Sensor_Curr_Angle_O : Constant  Value=0  OutDataTypeStr=single
  Str_Sensor_Curr_Angle_S : ArithShift
  Str_Sensor_Curr_Angle_Sub : Subsystem
  Str_Sensor_Curr_Angle_sat : Saturate  UpperLimit=900  LowerLimit=-900
  Str_Sensor_Curr_Anglecv : DataTypeConversion
  Str_Sensor_Curr_Angleinput2_Ad : Sum
  Str_Sensor_Curr_Angleinput2_C : Constant  Value=256
  Str_Sensor_Curr_Angleinput2_P : Product
  Str_Sensor_Curr_Anglesubcon : Sum  Inputs=+-
  Str_Sensor_Curr_Angle_Out : Outport
  wires:
  Str_Sensor_Curr_Angle_F/1 -> Str_Sensor_Curr_Angle_Ad/1
  Str_Sensor_Curr_Angle_O/1 -> Str_Sensor_Curr_Angle_Ad/2
  Str_Sensor_Curr_Angle_Ad/1 -> Str_Sensor_Curr_Angle_sat/1
  Str_Sensor_Curr_Angle_sat/1 -> Str_Sensor_Curr_Angle_Out/1
  Demux/2 -> Str_Sensor_Curr_Angleinput2_P/1
  Str_Sensor_Curr_Angleinput2_C/1 -> Str_Sensor_Curr_Angleinput2_P/2
  Str_Sensor_Curr_Angleinput2_P/1 -> Str_Sensor_Curr_Angleinput2_Ad/1
  Demux/3 -> Str_Sensor_Curr_Angleinput2_Ad/2
  Str_Sensor_Curr_Angleinput2_Ad/1 -> Str_Sensor_Curr_Angle_Sub/1(In1)
  Str_Sensor_Curr_Angle_Sub/1(Out1) -> Str_Sensor_Curr_Angle_Convert/1
  Str_Sensor_Curr_Angle_Convert/1 -> Str_Sensor_Curr_Angle_L/1
  Str_Sensor_Curr_Angle_L/1 -> Str_Sensor_Curr_Angle_S/1
  Str_Sensor_Curr_Angle_S/1 -> Str_Sensor_Curr_Anglecv/1
  Str_Sensor_Curr_Anglecv/1 -> Str_Sensor_Curr_AngleROP/1, Str_Sensor_Curr_Anglesubcon/2, Str_Sensor_Curr_AngleSW/3
  Str_Sensor_Curr_AngleConS/1 -> Str_Sensor_Curr_AngleCS/1, Str_Sensor_Curr_AngleCS1/1
  Str_Sensor_Curr_AngleCS1/1 -> Str_Sensor_Curr_AngleROP/2
  Str_Sensor_Curr_AngleCS/1 -> Str_Sensor_Curr_Anglesubcon/1
  Str_Sensor_Curr_Anglesubcon/1 -> Str_Sensor_Curr_AngleMinus/1
  Str_Sensor_Curr_AngleMinus/1 -> Str_Sensor_Curr_AngleSW/1
  Str_Sensor_Curr_AngleSW/1 -> Str_Sensor_Curr_Angle_F/1
  Str_Sensor_Curr_AngleROP/1 -> Str_Sensor_Curr_AngleSW/2
  input/1 -> Demux/1

== system FSAC2021/VCU_CAN_Read/PCANA(RES、AMI、MOTEC、BRAKE、STEER_SENSOR、IPC)/Str_Emergency  ==
  In1 : Inport
  function : TriggerPort  TriggerType=function-call
  Data Type Conversion{22..37} (16 alike) : DataTypeConversion  OutDataTypeStr=uint8
  MOTEC_EMERGENCY : Subsystem
  Str_UnderVolt_Warning_Out : Outport
  Str_System_Error_Out : Outport  Port=2
  Str_Spd_Over_Alam_Out : Outport  Port=3
  Str_PwrMod_TempHigh_Warning_Out : Outport  Port=4
  Str_PwrMod_TempHigh_Alarm_Out : Outport  Port=5
  Str_Para_Error_Out : Outport  Port=6
  Str_Overvolt_Warning_Out : Outport  Port=7
  Str_Over_TopCurr_Out : Outport  Port=8
  Str_Over_SpdError_Out : Outport  Port=9
  Str_Over_PosError_Out : Outport  Port=10
  Str_Limit_Pos_Alarm_Out : Outport  Port=11
  Str_I2t_Warning_Out : Outport  Port=12
  Str_I2t_Alarm_Out : Outport  Port=13
  Str_Flash_Error_Out : Outport  Port=14
  Str_Encoder_Error_Out : Outport  Port=15
  Str_Curr_Error_Fault_Out : Outport  Port=16
  wires:
  MOTEC_EMERGENCY/13(Str_I2t_Alarm_Out) -> Data Type Conversion34/1
  MOTEC_EMERGENCY/8(Str_Over_TopCurr_Out) -> Data Type Conversion29/1
  MOTEC_EMERGENCY/3(Str_Spd_Over_Alam_Out) -> Data Type Conversion24/1
  MOTEC_EMERGENCY/15(Str_Encoder_Error_Out) -> Data Type Conversion36/1
  MOTEC_EMERGENCY/5(Str_PwrMod_TempHigh_Alarm_Out) -> Data Type Conversion26/1
  MOTEC_EMERGENCY/9(Str_Over_SpdError_Out) -> Data Type Conversion30/1
  MOTEC_EMERGENCY/1(Str_UnderVolt_Warning_Out) -> Data Type Conversion22/1
  MOTEC_EMERGENCY/7(Str_Overvolt_Warning_Out) -> Data Type Conversion28/1
  MOTEC_EMERGENCY/11(Str_Limit_Pos_Alarm_Out) -> Data Type Conversion32/1
  MOTEC_EMERGENCY/2(Str_System_Error_Out) -> Data Type Conversion23/1
  MOTEC_EMERGENCY/14(Str_Flash_Error_Out) -> Data Type Conversion35/1
  MOTEC_EMERGENCY/4(Str_PwrMod_TempHigh_Warning_Out) -> Data Type Conversion25/1
  MOTEC_EMERGENCY/12(Str_I2t_Warning_Out) -> Data Type Conversion33/1
  MOTEC_EMERGENCY/10(Str_Over_PosError_Out) -> Data Type Conversion31/1
  MOTEC_EMERGENCY/16(Str_Curr_Error_Fault_Out) -> Data Type Conversion37/1
  MOTEC_EMERGENCY/6(Str_Para_Error_Out) -> Data Type Conversion27/1
  Data Type Conversion29/1 -> Str_Over_TopCurr_Out/1
  Data Type Conversion25/1 -> Str_PwrMod_TempHigh_Warning_Out/1
  Data Type Conversion27/1 -> Str_Para_Error_Out/1
  Data Type Conversion28/1 -> Str_Overvolt_Warning_Out/1
  Data Type Conversion30/1 -> Str_Over_SpdError_Out/1
  Data Type Conversion22/1 -> Str_UnderVolt_Warning_Out/1
  Data Type Conversion24/1 -> Str_Spd_Over_Alam_Out/1
  Data Type Conversion31/1 -> Str_Over_PosError_Out/1
  Data Type Conversion32/1 -> Str_Limit_Pos_Alarm_Out/1
  Data Type Conversion26/1 -> Str_PwrMod_TempHigh_Alarm_Out/1
  Data Type Conversion23/1 -> Str_System_Error_Out/1
  Data Type Conversion33/1 -> Str_I2t_Warning_Out/1
  Data Type Conversion35/1 -> Str_Flash_Error_Out/1
  Data Type Conversion36/1 -> Str_Encoder_Error_Out/1
  Data Type Conversion34/1 -> Str_I2t_Alarm_Out/1
  Data Type Conversion37/1 -> Str_Curr_Error_Fault_Out/1
  In1/1 -> MOTEC_EMERGENCY/1(input)

== system FSAC2021/VCU_CAN_Read/PCANA(RES、AMI、MOTEC、BRAKE、STEER_SENSOR、IPC)/Subsystem ==
  In1 : Inport
  In2 : Inport  Port=2
  In3 : Inport  Port=3
  Enable : EnablePort
  Data Type Conversion22 : DataTypeConversion
  Data Type Conversion23 : DataTypeConversion
  Data Type Conversion24 : DataTypeConversion
  Out1 : Outport
  Out2 : Outport  Port=2
  Out3 : Outport  Port=3
  wires:
  Data Type Conversion24/1 -> Out2/1
  Data Type Conversion23/1 -> Out3/1
  In1/1 -> Data Type Conversion22/1
  In2/1 -> Data Type Conversion24/1
  In3/1 -> Data Type Conversion23/1
  Data Type Conversion22/1 -> Out1/1

== system FSAC2021/VCU_CAN_Read/PCANB(BMS、DRIVE_MOTOR)/BMS_ALARM  ==
  In1 : Inport
  function : TriggerPort  TriggerType=function-call
  BMS_HCU_ALARM : Subsystem
  Data Type Conversion{38..62} (25 alike) : DataTypeConversion  OutDataTypeStr=uint8
  ALM_VCU_OFFLINE_Out : Outport
  ALM_PRECHRG_FAIL_Out : Outport  Port=2
  ALM_LEAK_OC_Out : Outport  Port=3
  ALM_HVREL_FAIL_Out : Outport  Port=4
  ALM_HALL_BREAK_Out : Outport  Port=5
  ALM_DSCH_OCT_Out : Outport  Port=6
  ALM_DSCH_OCS_Out : Outport  Port=7
  ALM_CHRG_OCT_Out : Outport  Port=8
  ALM_CHRG_OCS_Out : Outport  Port=9
  ALM_BSU_OFFLINE_Out : Outport  Port=10
  ALM_BSU_FAULT_Out : Outport  Port=11
  ALM_BMU_FAIL_Out : Outport  Port=12
  ALM_BATT_UC_Out : Outport  Port=13
  ALM_BATT_OC_Out : Outport  Port=14
  ALM_AUX_FAIL_Out : Outport  Port=15
  ALM_BATT_UV_Out : Outport  Port=16
  ALM_BATT_OV_Out : Outport  Port=17
  ALM_BATT_DT_Out : Outport  Port=18
  ALM_BATT_DV_Out : Outport  Port=19
  ALM_CELL_TBK_Out : Outport  Port=20
  ALM_CELL_IBK_Out : Outport  Port=21
  ALM_CELL_UT_Out : Outport  Port=22
  ALM_CELL_OT_Out : Outport  Port=23
  ALM_CELL_UV_Out : Outport  Port=24
  ALM_CELL_OV_Out : Outport  Port=25
  wires:
  BMS_HCU_ALARM/22(ALM_CELL_UT_Out) -> Data Type Conversion59/1
  BMS_HCU_ALARM/25(ALM_CELL_OV_Out) -> Data Type Conversion62/1
  BMS_HCU_ALARM/20(ALM_CELL_TBK_Out) -> Data Type Conversion57/1
  BMS_HCU_ALARM/14(ALM_BATT_OC_Out) -> Data Type Conversion51/1
  BMS_HCU_ALARM/24(ALM_CELL_UV_Out) -> Data Type Conversion61/1
  BMS_HCU_ALARM/21(ALM_CELL_IBK_Out) -> Data Type Conversion58/1
  BMS_HCU_ALARM/23(ALM_CELL_OT_Out) -> Data Type Conversion60/1
  BMS_HCU_ALARM/1(ALM_VCU_OFFLINE_Out) -> Data Type Conversion38/1
  BMS_HCU_ALARM/19(ALM_BATT_DV_Out) -> Data Type Conversion56/1
  BMS_HCU_ALARM/6(ALM_DSCH_OCT_Out) -> Data Type Conversion43/1
  BMS_HCU_ALARM/17(ALM_BATT_OV_Out) -> Data Type Conversion54/1
  BMS_HCU_ALARM/18(ALM_BATT_DT_Out) -> Data Type Conversion55/1
  BMS_HCU_ALARM/7(ALM_DSCH_OCS_Out) -> Data Type Conversion44/1
  BMS_HCU_ALARM/16(ALM_BATT_UV_Out) -> Data Type Conversion53/1
  BMS_HCU_ALARM/13(ALM_BATT_UC_Out) -> Data Type Conversion50/1
  BMS_HCU_ALARM/15(ALM_AUX_FAIL_Out) -> Data Type Conversion52/1
  BMS_HCU_ALARM/8(ALM_CHRG_OCT_Out) -> Data Type Conversion45/1
  Data Type Conversion38/1 -> ALM_VCU_OFFLINE_Out/1
  BMS_HCU_ALARM/5(ALM_HALL_BREAK_Out) -> Data Type Conversion42/1
  BMS_HCU_ALARM/10(ALM_BSU_OFFLINE_Out) -> Data Type Conversion47/1
  BMS_HCU_ALARM/12(ALM_BMU_FAIL_Out) -> Data Type Conversion49/1
  BMS_HCU_ALARM/2(ALM_PRECHRG_FAIL_Out) -> Data Type Conversion40/1
  BMS_HCU_ALARM/3(ALM_LEAK_OC_Out) -> Data Type Conversion39/1
  BMS_HCU_ALARM/4(ALM_HVREL_FAIL_Out) -> Data Type Conversion41/1
  BMS_HCU_ALARM/11(ALM_BSU_FAULT_Out) -> Data Type Conversion48/1
  BMS_HCU_ALARM/9(ALM_CHRG_OCS_Out) -> Data Type Conversion46/1
  Data Type Conversion47/1 -> ALM_BSU_OFFLINE_Out/1
  Data Type Conversion41/1 -> ALM_HVREL_FAIL_Out/1
  Data Type Conversion43/1 -> ALM_HALL_BREAK_Out/1
  Data Type Conversion42/1 -> ALM_DSCH_OCT_Out/1
  Data Type Conversion45/1 -> ALM_CHRG_OCT_Out/1
  Data Type Conversion40/1 -> ALM_PRECHRG_FAIL_Out/1
  Data Type Conversion39/1 -> ALM_LEAK_OC_Out/1
  Data Type Conversion46/1 -> ALM_CHRG_OCS_Out/1
  Data Type Conversion44/1 -> ALM_DSCH_OCS_Out/1
  Data Type Conversion50/1 -> ALM_BATT_UC_Out/1
  Data Type Conversion51/1 -> ALM_BATT_OC_Out/1
  Data Type Conversion53/1 -> ALM_BATT_UV_Out/1
  Data Type Conversion54/1 -> ALM_BATT_OV_Out/1
  Data Type Conversion52/1 -> ALM_AUX_FAIL_Out/1
  Data Type Conversion48/1 -> ALM_BSU_FAULT_Out/1
  Data Type Conversion55/1 -> ALM_BATT_DT_Out/1
  Data Type Conversion56/1 -> ALM_BATT_DV_Out/1
  Data Type Conversion49/1 -> ALM_BMU_FAIL_Out/1
  Data Type Conversion61/1 -> ALM_CELL_UV_Out/1
  Data Type Conversion58/1 -> ALM_CELL_IBK_Out/1
  Data Type Conversion60/1 -> ALM_CELL_OT_Out/1
  Data Type Conversion59/1 -> ALM_CELL_UT_Out/1
  Data Type Conversion62/1 -> ALM_CELL_OV_Out/1
  Data Type Conversion57/1 -> ALM_CELL_TBK_Out/1
  In1/1 -> BMS_HCU_ALARM/1(input)
